simulink model "Control_SMC_con_Perturbaciones"  (R2025b)
settings: Solver=ode45  StartTime=0.0  StopTime=12  RelTol=1e-3
settings Model: Creator=Carlo  LastModifiedBy=Carlo
settings DataIOCC: SaveState=on

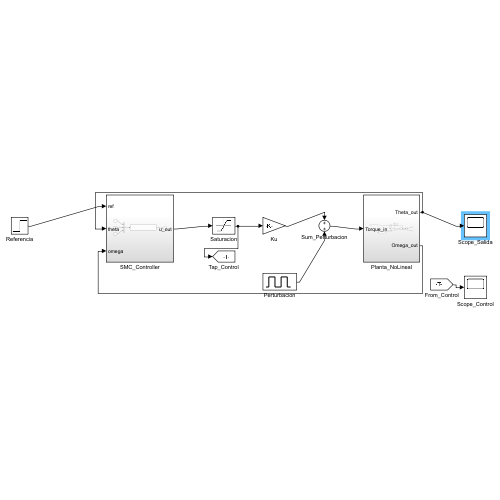
[thumbnail: Simulink's stored preview of the top-level diagram]
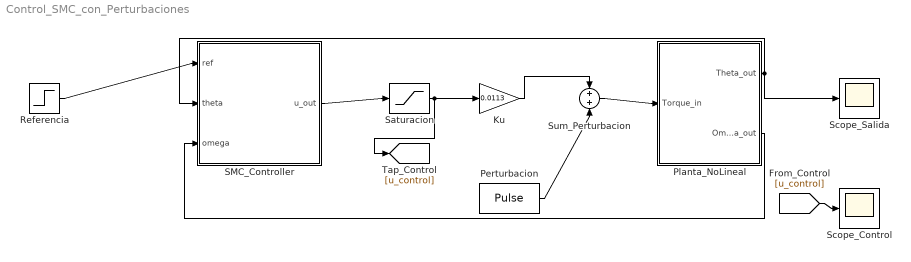
== system Control_SMC_con_Perturbaciones ==
  Ku : Gain  Gain=0.0113
  Perturbacion : DiscretePulseGenerator  PulseType=Time based  Amplitude=0.002  Period=3  PulseWidth=20
  Planta_NoLineal : Subsystem
  Referencia : Step  Time=0  After=0.87266  SampleTime=0
  SMC_Controller : Subsystem
  Saturacion : Saturate  UpperLimit=1  LowerLimit=-1
  Scope_Control : Scope
  Scope_Salida : Scope
      settings: ActiveDisplayYMinimum=0.870945595272495  ActiveDisplayYMaximum=0.88808964254754452
  Sum_Perturbacion : Sum
  wires:
  Referencia/1 -> SMC_Controller/1(ref)
  SMC_Controller/1(u_out) -> Saturacion/1
  Saturacion/1 -> Ku/1, [u_control]
  Ku/1 -> Sum_Perturbacion/1
  Perturbacion/1 -> Sum_Perturbacion/2
  Sum_Perturbacion/1 -> Planta_NoLineal/1(Torque_in)
  Planta_NoLineal/1(Theta_out) -> Scope_Salida/1, SMC_Controller/2(theta)
  Planta_NoLineal/2(Omega_out) -> SMC_Controller/3(omega)
  [u_control] -> Scope_Control/1

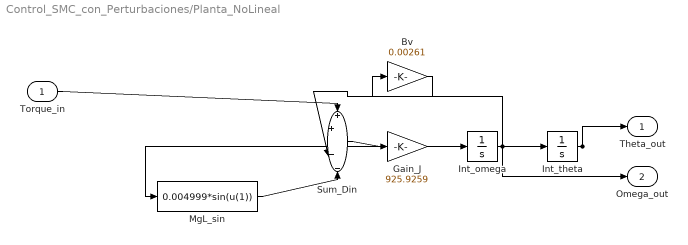
== system Control_SMC_con_Perturbaciones/Planta_NoLineal ==
  Torque_in : Inport
  Bv : Gain  Gain=0.00261
  Gain_J : Gain  Gain=925.9259
  Int_omega : Integrator
  Int_theta : Integrator  InitialCondition=0.87266
  MgL_sin : Fcn  Expr=0.004999*sin(u(1))
  Sum_Din : Sum  Inputs=++--
  Theta_out : Outport
  Omega_out : Outport  Port=2
  wires:
  Torque_in/1 -> Sum_Din/1
  Sum_Din/1 -> Gain_J/1
  Gain_J/1 -> Int_omega/1
  Int_omega/1 -> Int_theta/1, Omega_out/1, Bv/1
  Int_theta/1 -> Theta_out/1, MgL_sin/1
  MgL_sin/1 -> Sum_Din/4
  Bv/1 -> Sum_Din/3

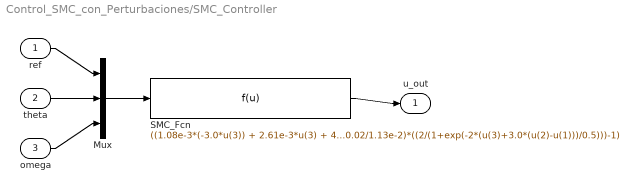
== system Control_SMC_con_Perturbaciones/SMC_Controller ==
  ref : Inport
  theta : Inport  Port=2
  omega : Inport  Port=3
  Mux : Mux  Inputs=3
  SMC_Fcn : Fcn  Expr=((1.08e-3*(-3.0*u(3)) + 2.61e-3*u(3) + 4.999e-3*sin(u(2)))/1.13e-2) - (0.02/1.13e-2)*((2/(1+exp(-2*(u(3)+3.0*(u(2)-u(1)))/0.5)))-1)
  u_out : Outport
  wires:
  ref/1 -> Mux/1
  theta/1 -> Mux/2
  omega/1 -> Mux/3
  Mux/1 -> SMC_Fcn/1
  SMC_Fcn/1 -> u_out/1
